simulink model "ctg_ut"  (Simulink 8.1)
settings: Solver=FixedStepDiscrete  StartTime=0.0  StopTime=Inf  FixedStep=0.005  RelTol=1e-3
PostLoadFcn:
  | , if any(exist('dsrtsu_mdlpostloadfcn', 'file') == [2, 3, 6]), try dsrtsu_mdlpostloadfcn('Execute', bdroot); catch fprintf('Error in PostLoadFcn (dsrtsu_mdlpostloadfcn) for model "%s":\n %s\n', bdroot, lasterr); end, end,
libraries: siltestlib x6, ctg x1
settings Model: DSRTSU_INTERNAL_RTI_VER=450  DSRTSU_INTERNAL_RTI_TYPE=rti1401  RTICANMMDATA=struct('GeneralSetupData',struct('modelroot','D:\ELN150201_TAIWAN\trunk\AdasDragon\software\sw_development\arch\app\acc','generalsettings',struct('filesettings',struct('destfolder',struct('Name','RTICANMM_FILES','Check',1),'buildfolder',struct('Name','.','Check',1),'AbsDestfolder',struct('Name','D:\ELN150201_TAIWAN\trunk\AdasDragon\software\sw_development\arch\app\acc\RTICANMM_FILES'),'AbsBuildfolder',struct('Name','D:\ELN150201_TAIWAN\trunk\AdasDragon\software\sw_development\arch\app\acc'))),'options',struct('addpaths',1,'rmpaths',1,'addtrcexclusion',logical(1),'cannavigator',struct('checkmonitoring',0),'show_usrtrc',0,'use_usrtrc',0),'advanced',struct('options',[1 1 1 1 1 1 1 1 1 1 1 1 1 1 1 1 1 1 1 1 1 1 1 1 1 1 1 1 1 1 1 1 1 1 1 1 1 1 1 1 1 1 1 1 1 1 1 1 1 1 1 1 1 1 1 1 1 1 1 1 1 1 1 1 1 1 1 1 1 1 1 1 1 1 1 1 1 1 1 1 1 1 1 1 1 1 1 1 1 1 1 1 1 1 1 1 1 1 1 1]),'MPSetup',{{}},'modelname','ctg_ut','block','ctg_ut'))  DSRTSU_INTERNAL_RTIFPGA=40  Creator=idiada  LastModifiedBy=AT015555  BufferReuse=off
settings DataIOCC: SignalLoggingSaveFormat=Dataset
settings OptimizationCC: BlockReduction=off  OptimizeBlockIOStorage=off  BufferReuse=off  ExpressionFolding=off  ExpressionDepthLimit=128  LocalBlockOutputs=off
settings DebuggingCC: FcnCallInpInsideContextMsg=EnableAllAsError
settings HardwareCC: TargetHWDeviceType=Generic->Custom
settings RTWCC: SystemTargetFile=rti1401.tlc  MakeCommand=make_rti  TemplateMakefile=rti1401.tmf  Description=dSPACE DS1401 Hardware Platform  ProcessScript=rti1401_make_rtw_hook
settings STFCustomTargetCC: CodeReplacementLibrary=ANSI_C  ParMdlRefBuildCompliant=on  GeneratePreprocessorConditionals=Disable all  MatFileLogging=on  SystemTargetFile=rti1401.tlc
settings GRTTargetCC: CompOptLevelCompliant=off  ConcurrentExecutionCompliant=off  ExtModeMexFile=noextcomm
settings CustomProperty: DataType=RTWOptions_EnumType_C__Program Files (x86)_dSPACE RCPHIL 2014-B_MATLAB_RTI_RTI1401_TLC_rti1401_1InitialSimState  Value=RUN
settings EnumStrPairs: String=RUN

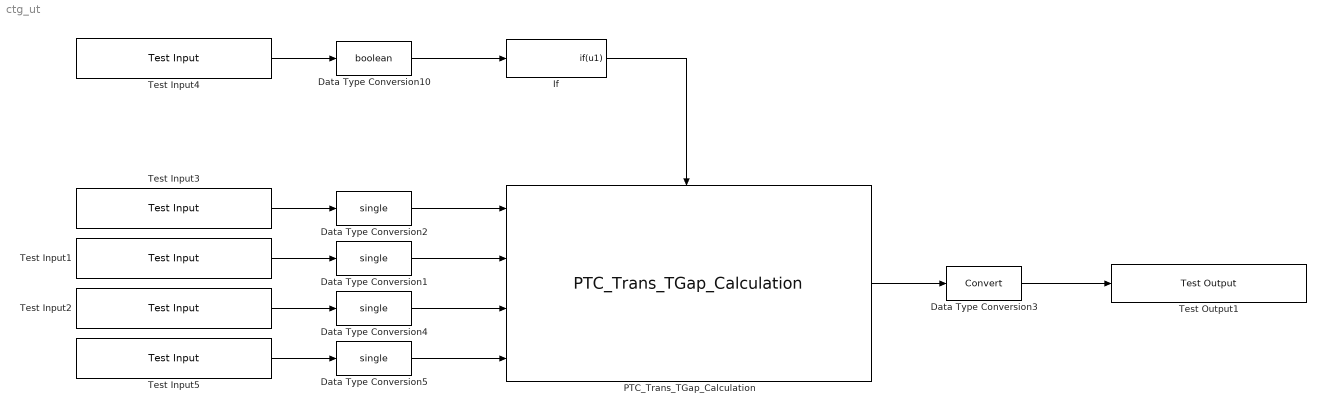
== system ctg_ut ==
  Data Type Conversion{1..2,4..5} (4 alike) : DataTypeConversion  OutDataTypeStr=single
  Data Type Conversion10 : DataTypeConversion  OutDataTypeStr=boolean
  Data Type Conversion3 : DataTypeConversion
  If : If  IfExpression=u1  ShowElse=off
  PTC_Trans_TGap_Calculation : ctg/PTC_Trans_TGap_Calculation
  Test Input1 : siltestlib/Test Input  varname=VIFO_ACCVehClearance_m  sampletime=0.005
  Test Input2 : siltestlib/Test Input  varname=VACC_DesiredDistance_m  sampletime=0.005
  Test Input3 : siltestlib/Test Input  varname=VDINR_VehSpd_mps  sampletime=0.005
  Test Input4 : siltestlib/Test Input  varname=Block_Enable_Input  sampletime=0.005
  Test Input5 : siltestlib/Test Input  varname=VIFO_ACCTargetVehRelSpeedX_mps  sampletime=0.005
  Test Output1 : siltestlib/Test Output  varname=VACC_TransTGapPTC_flg  sampletime=-1
  wires:
  Test Input4/1 -> Data Type Conversion10/1
  Data Type Conversion10/1 -> If/1
  If/1 -> PTC_Trans_TGap_Calculation/Action
  Test Input1/1 -> Data Type Conversion1/1
  Data Type Conversion1/1 -> PTC_Trans_TGap_Calculation/2
  Test Input2/1 -> Data Type Conversion4/1
  Data Type Conversion4/1 -> PTC_Trans_TGap_Calculation/3
  Data Type Conversion3/1 -> Test Output1/1
  PTC_Trans_TGap_Calculation/1 -> Data Type Conversion3/1
  Test Input3/1 -> Data Type Conversion2/1
  Data Type Conversion2/1 -> PTC_Trans_TGap_Calculation/1
  Test Input5/1 -> Data Type Conversion5/1
  Data Type Conversion5/1 -> PTC_Trans_TGap_Calculation/4
